simulink model "tankSim"  (R2025a)
settings: Solver=VariableStepAuto  StartTime=0.0  StopTime=100  RelTol=1e-3
values from neighbouring files (symbols this model uses):
  A = result_table.Apogee_m    [runFlightSimSweep.m]    (also in runTankSim.m = 0.389151343947)
  B_liq = 1.2e-3    (= 0.0012)    [runTankSim.m]
  B_vap = 3.33e-3    (= 0.00333)    [runTankSim.m]
  C_liq = 0.021    [runTankSim.m]
  c_p = 0.88    [runTankSim.m]
  C_vap = 0.021    [runTankSim.m]
  g = 9.79346    [runTankSim.m]
  k_liq = 0.109    [runTankSim.m]
  k_vap = 0.0152    [runTankSim.m]
  L = 2*r    (= 0.2032)    [runTankSim.m]
  m_tot0 = V_tank*(x_test/py.CoolProp.CoolProp.PropsSI('D', 'T', T, 'Q', 1, 'NitrousOxide') + (1-x_test)/py.CoolProp.CoolProp.PropsSI('D', 'T', T, 'Q', 0, 'NitrousOxide'))^(-1)    [runTankSim.m]
  mu = 1.48e-5    (= 1.48e-05)    [runTankSim.m]
  n_liq = 0.4    [runTankSim.m]
  n_vap = 0.4    [runTankSim.m]
  p_amb = 101325    [runTankSim.m]
  U_tot0 = ((1-x_test)*py.CoolProp.CoolProp.PropsSI('H', 'T', T, 'Q', 0, 'NitrousOxide')+x_test*py.CoolProp.CoolProp.PropsSI('H', 'T', T, 'Q', 1, 'NitrousOxide'))*m_tot0    [runTankSim.m]
  V_tank = pi * r^2 * H    (= 0.0164740735604)    [runTankSim.m]
  x_full = 0.12    [runTankSim.m]
libraries: simulink x1
settings Model: Creator=Nick  LastModifiedBy=Nick

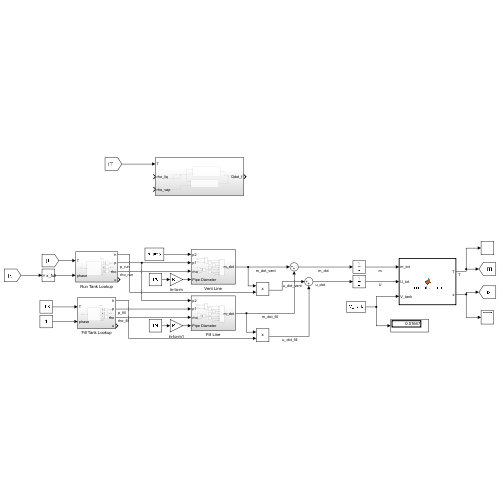
[thumbnail: Simulink's stored preview of the top-level diagram]
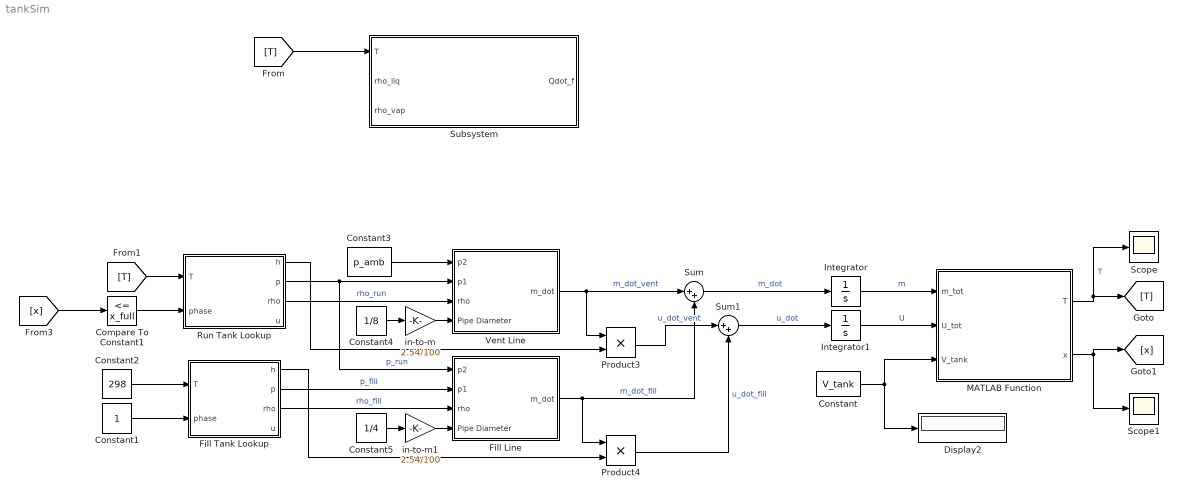
== system tankSim ==
  Compare To Constant1 : simulink/Logic and Bit Operations/Compare To Constant  relop=<=  const=x_full  OutDataTypeStr=boolean
  Constant : Constant  Value=V_tank
  Constant1 : Constant
  Constant2 : Constant  Value=298
  Constant3 : Constant  Value=p_amb
  Constant4 : Constant  Value=1/8
  Constant5 : Constant  Value=1/4
  Display2 : Display
  Fill Line : Subsystem
  Fill Tank Lookup : Subsystem
  Integrator : Integrator  InitialCondition=m_tot0
  Integrator1 : Integrator  InitialCondition=U_tot0
  MATLAB Function : MATLAB Function  TreatAsAtomicUnit=on
  Product3 : Product
  Product4 : Product
  Run Tank Lookup : Subsystem
  Scope : Scope
      settings: ActiveDisplayYMinimum=292.5382899506879  ActiveDisplayYMaximum=313.86878460753451
  Scope1 : Scope
      settings: ActiveDisplayYMinimum=-2.6427364376879452  ActiveDisplayYMaximum=4.78271456468242
  Subsystem : Subsystem
  Sum : Sum  Inputs=|++
  Sum1 : Sum  Inputs=|++
  Vent Line : Subsystem
  in-to-m : Gain  Gain=2.54/100
  in-to-m1 : Gain  Gain=2.54/100
  wires:
  [T] -> Subsystem/1(T)
  Constant2/1 -> Fill Tank Lookup/1(T)
  Constant1/1 -> Fill Tank Lookup/2(phase)
  Vent Line/1(m_dot) -> Product3/1, Sum/1  "m_dot_vent"
  [T] -> Run Tank Lookup/1(T)
  Compare To Constant1/1 -> Run Tank Lookup/2(phase)
  [x] -> Compare To Constant1/1
  Fill Line/1(m_dot) -> Sum/2, Product4/1  "m_dot_fill"
  Product3/1 -> Sum1/1  "u_dot_vent"
  Product4/1 -> Sum1/2  "u_dot_fill"
  Fill Tank Lookup/3(rho) -> Fill Line/3(rho)  "rho_fill"
  Run Tank Lookup/3(rho) -> Vent Line/3(rho)  "rho_run"
  Constant/1 -> MATLAB Function/3(V_tank), Display2/1
  MATLAB Function/1(T) -> Scope/1, [T]  "T"
  MATLAB Function/2(x) -> [x], Scope1/1
  Integrator/1 -> MATLAB Function/1(m_tot)  "m"
  Integrator1/1 -> MATLAB Function/2(U_tot)  "U"
  Sum/1 -> Integrator/1  "m_dot"
  Sum1/1 -> Integrator1/1  "u_dot"
  Constant4/1 -> in-to-m/1
  in-to-m/1 -> Vent Line/4(Pipe Diameter)
  Constant5/1 -> in-to-m1/1
  in-to-m1/1 -> Fill Line/4(Pipe Diameter)
  Constant3/1 -> Vent Line/1(p2)
  Run Tank Lookup/2(p) -> Fill Line/1(p2), Vent Line/2(p1)  "p_run"
  Fill Tank Lookup/2(p) -> Fill Line/2(p1)  "p_fill"
  Run Tank Lookup/1(h) -> Product3/2
  Fill Tank Lookup/1(h) -> Product4/2

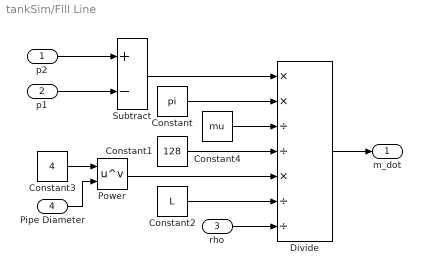
== system tankSim/Fill Line ==
  p2 : Inport
  p1 : Inport  Port=2
  rho : Inport  Port=3
  Pipe Diameter : Inport  Port=4
  Constant : Constant  Value=pi
  Constant1 : Constant  Value=128
  Constant2 : Constant  Value=L
  Constant3 : Constant  Value=4
  Constant4 : Constant  Value=mu
  Divide : Product  Inputs=**//*//
  Power : Math  Operator=pow
  Subtract : Sum  Inputs=+-
  m_dot : Outport
  wires:
  Subtract/1 -> Divide/1
  p1/1 -> Subtract/2
  p2/1 -> Subtract/1
  Constant/1 -> Divide/2
  Constant1/1 -> Divide/4
  Constant2/1 -> Divide/6
  rho/1 -> Divide/7
  Divide/1 -> m_dot/1
  Constant4/1 -> Divide/3
  Power/1 -> Divide/5
  Constant3/1 -> Power/1
  Pipe Diameter/1 -> Power/2

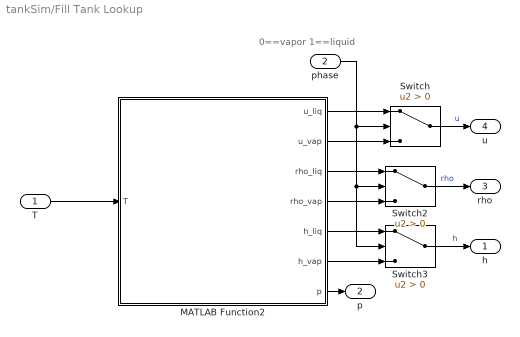
== system tankSim/Fill Tank Lookup ==
  note: 0==vapor
      | 1==liquid
  T : Inport
  phase : Inport  Port=2
  MATLAB Function2 : MATLAB Function  TreatAsAtomicUnit=on
  Switch : Switch  Criteria=u2 > Threshold  SaturateOnIntegerOverflow=off  InputSameDT=off
  Switch2 : Switch  Criteria=u2 > Threshold  SaturateOnIntegerOverflow=off  InputSameDT=off
  Switch3 : Switch  Criteria=u2 > Threshold  SaturateOnIntegerOverflow=off  InputSameDT=off
  h : Outport
  p : Outport  Port=2
  rho : Outport  Port=3
  u : Outport  Port=4
  wires:
  MATLAB Function2/5(h_liq) -> Switch3/1
  phase/1 -> Switch/2, Switch3/2, Switch2/2
  MATLAB Function2/2(u_vap) -> Switch/3
  MATLAB Function2/4(rho_vap) -> Switch2/3
  Switch2/1 -> rho/1  "rho"
  MATLAB Function2/6(h_vap) -> Switch3/3
  MATLAB Function2/1(u_liq) -> Switch/1
  T/1 -> MATLAB Function2/1(T)
  MATLAB Function2/3(rho_liq) -> Switch2/1
  Switch3/1 -> h/1  "h"
  MATLAB Function2/7(p) -> p/1
  Switch/1 -> u/1  "u"

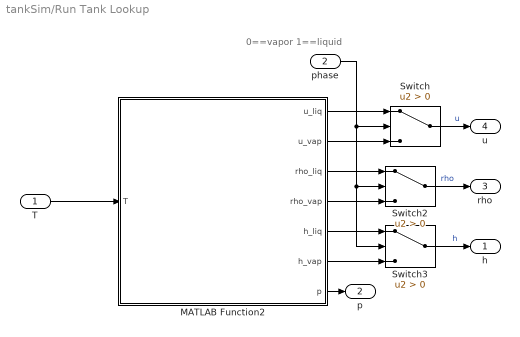
== system tankSim/Run Tank Lookup ==
  note: 0==vapor
      | 1==liquid
  T : Inport
  phase : Inport  Port=2
  MATLAB Function2 : MATLAB Function  TreatAsAtomicUnit=on
  Switch : Switch  Criteria=u2 > Threshold  SaturateOnIntegerOverflow=off  InputSameDT=off
  Switch2 : Switch  Criteria=u2 > Threshold  SaturateOnIntegerOverflow=off  InputSameDT=off
  Switch3 : Switch  Criteria=u2 > Threshold  SaturateOnIntegerOverflow=off  InputSameDT=off
  h : Outport
  p : Outport  Port=2
  rho : Outport  Port=3
  u : Outport  Port=4
  wires:
  Switch/1 -> u/1  "u"
  MATLAB Function2/7(p) -> p/1
  Switch3/1 -> h/1  "h"
  MATLAB Function2/3(rho_liq) -> Switch2/1
  T/1 -> MATLAB Function2/1(T)
  MATLAB Function2/1(u_liq) -> Switch/1
  MATLAB Function2/6(h_vap) -> Switch3/3
  Switch2/1 -> rho/1  "rho"
  MATLAB Function2/4(rho_vap) -> Switch2/3
  MATLAB Function2/2(u_vap) -> Switch/3
  phase/1 -> Switch2/2, Switch3/2, Switch/2
  MATLAB Function2/5(h_liq) -> Switch3/1

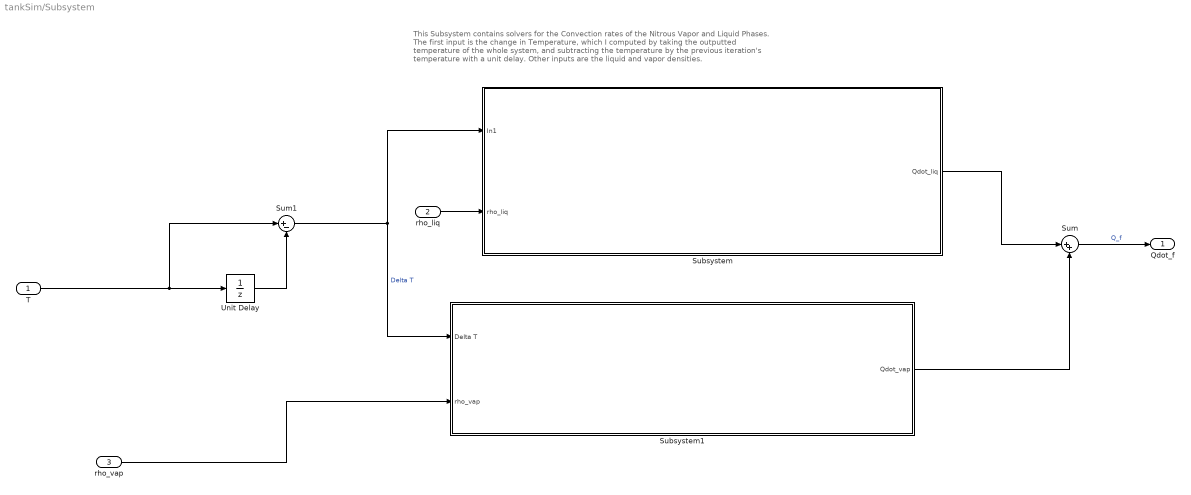
== system tankSim/Subsystem ==
  note: This Subsystem contains solvers for the Convection rates of the Nitrous Vapor and Liquid Phases. The first input is the change in Temperature, which I computed by taking the outputted temperature of the whole system, and subtracting the temperature by the previous iteration's temperature with a unit delay. Other inputs are the liquid and vapor densities.
  T : Inport
  rho_liq : Inport  Port=2
  rho_vap : Inport  Port=3
  Subsystem : Subsystem
  Subsystem1 : Subsystem
  Sum : Sum  Inputs=|++
  Sum1 : Sum  Inputs=|+-
  Unit Delay : UnitDelay  SampleTime=-1  HasFrameUpgradeWarning=on
  Qdot_f : Outport
  wires:
  Unit Delay/1 -> Sum1/2
  T/1 -> Sum1/1, Unit Delay/1
  Sum1/1 -> Subsystem1/1(Delta T), Subsystem/1(In1)  "Delta T"
  rho_liq/1 -> Subsystem/2(rho_liq)
  Subsystem/1(Qdot_liq) -> Sum/1
  rho_vap/1 -> Subsystem1/2(rho_vap)
  Subsystem1/1(Qdot_vap) -> Sum/2
  Sum/1 -> Qdot_f/1  "Q_f"

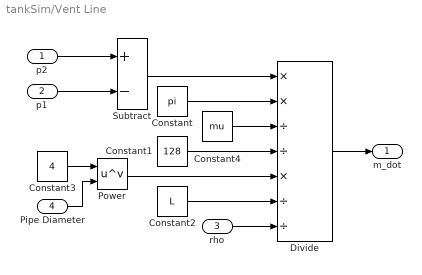
== system tankSim/Vent Line ==
  p2 : Inport
  p1 : Inport  Port=2
  rho : Inport  Port=3
  Pipe Diameter : Inport  Port=4
  Constant : Constant  Value=pi
  Constant1 : Constant  Value=128
  Constant2 : Constant  Value=L
  Constant3 : Constant  Value=4
  Constant4 : Constant  Value=mu
  Divide : Product  Inputs=**//*//
  Power : Math  Operator=pow
  Subtract : Sum  Inputs=+-
  m_dot : Outport
  wires:
  Subtract/1 -> Divide/1
  p1/1 -> Subtract/2
  p2/1 -> Subtract/1
  Constant/1 -> Divide/2
  Constant1/1 -> Divide/4
  Constant2/1 -> Divide/6
  rho/1 -> Divide/7
  Divide/1 -> m_dot/1
  Constant4/1 -> Divide/3
  Power/1 -> Divide/5
  Constant3/1 -> Power/1
  Pipe Diameter/1 -> Power/2

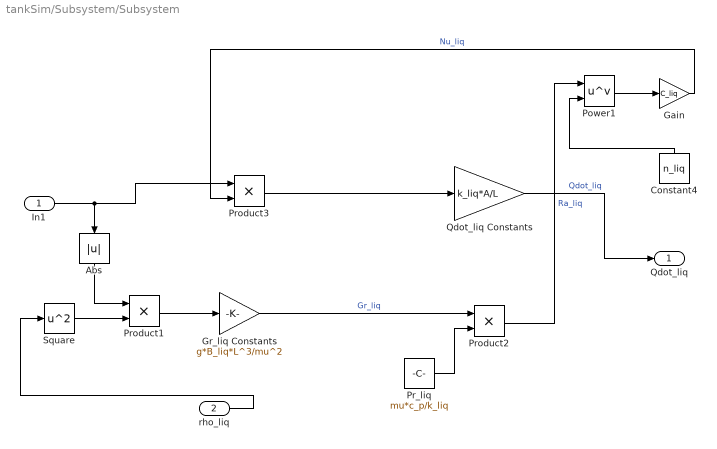
== system tankSim/Subsystem/Subsystem ==
  In1 : Inport
  rho_liq : Inport  Port=2
  Abs : Abs  SaturateOnIntegerOverflow=off
  Constant4 : Constant  Value=n_liq
  Gain : Gain  Gain=C_liq
  Gr_liq Constants : Gain  Gain=g*B_liq*L^3/mu^2
  Power1 : Math  Operator=pow
  Pr_liq : Constant  Value=mu*c_p/k_liq
  Product1 : Product
  Product2 : Product
  Product3 : Product
  Qdot_liq Constants : Gain  Gain=k_liq*A/L
  Square : Math  Operator=square
  Qdot_liq : Outport
  wires:
  Qdot_liq Constants/1 -> Qdot_liq/1  "Qdot_liq"
  Product2/1 -> Power1/1  "Ra_liq"
  Pr_liq/1 -> Product2/2
  In1/1 -> Product3/1, Abs/1
  Gain/1 -> Product3/2  "Nu_liq"
  Gr_liq Constants/1 -> Product2/1  "Gr_liq"
  Product1/1 -> Gr_liq Constants/1
  Square/1 -> Product1/2
  Power1/1 -> Gain/1
  rho_liq/1 -> Square/1
  Constant4/1 -> Power1/2
  Product3/1 -> Qdot_liq Constants/1
  Abs/1 -> Product1/1

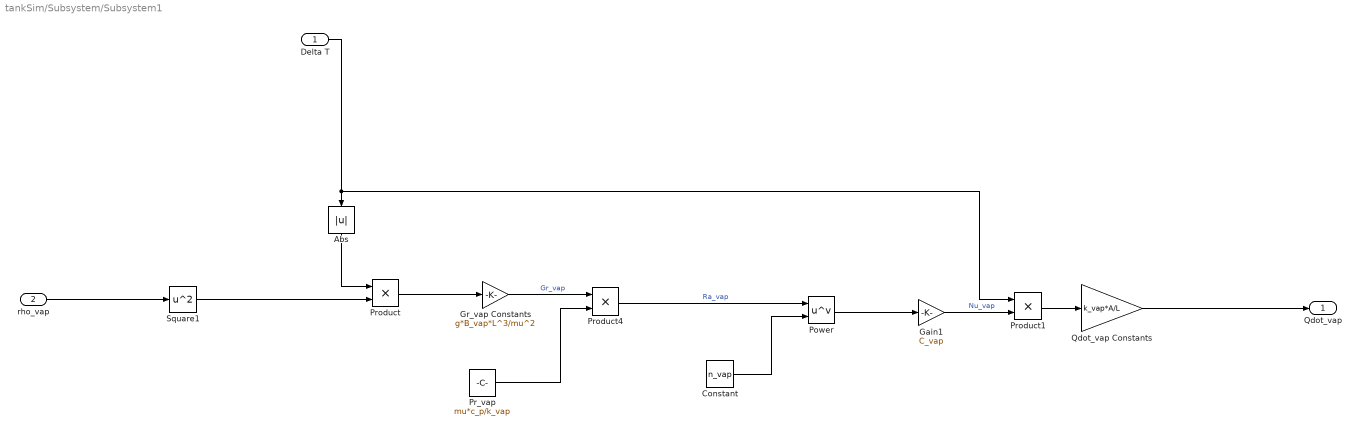
== system tankSim/Subsystem/Subsystem1 ==
  Delta T : Inport
  rho_vap : Inport  Port=2
  Abs : Abs  SaturateOnIntegerOverflow=off
  Constant : Constant  Value=n_vap
  Gain1 : Gain  Gain=C_vap
  Gr_vap Constants : Gain  Gain=g*B_vap*L^3/mu^2
  Power : Math  Operator=pow
  Pr_vap : Constant  Value=mu*c_p/k_vap
  Product : Product
  Product1 : Product
  Product4 : Product
  Qdot_vap Constants : Gain  Gain=k_vap*A/L
  Square1 : Math  Operator=square
  Qdot_vap : Outport
  wires:
  rho_vap/1 -> Square1/1
  Qdot_vap Constants/1 -> Qdot_vap/1
  Gain1/1 -> Product1/2  "Nu_vap"
  Square1/1 -> Product/2
  Abs/1 -> Product/1
  Delta T/1 -> Product1/1, Abs/1
  Product4/1 -> Power/1  "Ra_vap"
  Pr_vap/1 -> Product4/2
  Power/1 -> Gain1/1
  Product1/1 -> Qdot_vap Constants/1
  Constant/1 -> Power/2
  Product/1 -> Gr_vap Constants/1
  Gr_vap Constants/1 -> Product4/1  "Gr_vap"

== matlab function tankSim/Run Tank Lookup/MATLAB Function2 ==
  data: T input; u_liq output; u_vap output; rho_liq output; rho_vap output; h_liq output; h_vap output; p output
function [u_liq,u_vap,rho_liq,rho_vap,h_liq,h_vap,p] = CoolPropLookup(T)
lookup = load('CoolPropLookup.mat');
u_liq = interp1(lookup.T_range, lookup.u_liq, T,"linear");
u_vap = interp1(lookup.T_range, lookup.u_vap, T,"linear");
rho_liq = interp1(lookup.T_range, lookup.rho_liq, T,"linear");
rho_vap = interp1(lookup.T_range, lookup.rho_vap, T,"linear");
h_liq = interp1(lookup.T_range, lookup.h_liq, T,"linear");
h_vap = interp1(lookup.T_range, lookup.h_vap, T,"linear");
p = interp1(lookup.T_range, lookup.p, T, "linear");

== matlab function tankSim/MATLAB Function ==
  data: m_tot input; T output; U_tot input; V_tank input; x output
function [T, x]= calculate_state(m_tot, U_tot, V_tank)
    lookup = load('CoolPropLookup.mat');
    T_range = lookup.T_range;
    u_liq = lookup.u_liq;
    u_vap = lookup.u_vap;
    rho_vap = lookup.rho_vap;
    rho_liq = lookup.rho_liq;
    h_vap = lookup.h_vap;
    h_liq = lookup.h_liq;
    p = lookup.p;
    % Resduals anonymous function given U_tot m_tot and V_tank
    residual_function = @(x) [(1-x(1)) * interp1(lookup.T_range, lookup.u_liq, x(2), "linear") + x(1) * interp1(lookup.T_range, lookup.u_vap, x(2), "linear")-U_tot/m_tot;
             (x(1)/interp1(lookup.T_range, lookup.rho_vap, x(2), "linear") + (1-x(1))/interp1(lookup.T_range, lookup.rho_liq, x(2), "linear"))*m_tot-V_tank];
    % Innitial guess
    x0 = [0.5; 298];
    % solve
    options = optimoptions('fsolve', 'Algorithm', 'levenberg-marquardt', 'Display', 'iter');
    [solution,fval] = fsolve(residual_function,x0,options);
    x = solution(1);
    T = solution(2);

== matlab function tankSim/Fill Tank Lookup/MATLAB Function2 ==
  data: T input; u_liq output; u_vap output; rho_liq output; rho_vap output; h_liq output; h_vap output; p output
function [u_liq,u_vap,rho_liq,rho_vap,h_liq,h_vap,p] = CoolPropLookup(T)
lookup = load('CoolPropLookup.mat');
u_liq = interp1(lookup.T_range, lookup.u_liq, T,"linear");
u_vap = interp1(lookup.T_range, lookup.u_vap, T,"linear");
rho_liq = interp1(lookup.T_range, lookup.rho_liq, T,"linear");
rho_vap = interp1(lookup.T_range, lookup.rho_vap, T,"linear");
h_liq = interp1(lookup.T_range, lookup.h_liq, T,"linear");
h_vap = interp1(lookup.T_range, lookup.h_vap, T,"linear");
p = interp1(lookup.T_range, lookup.p, T, "linear");
